simulink model "sowavedec2imaq"  (R2012a)
settings: Solver=FixedStepDiscrete  StartTime=0.0  StopTime=inf  RelTol=1e-3
undefined symbols (not defined in the file or in its folder): jet, none, videoinput
libraries: imaqlib x1, visionsinks x1
settings Model: ExtModeTrigDuration=100  Creator=harashin  LastModifiedBy=Shogo
settings DataIOCC: LimitDataPoints=on  SaveFormat=Array  ReturnWorkspaceOutputs=off
settings OptimizationCC: ExpressionDepthLimit=2147483647  OptimizeModelRefInitCode=on  LifeSpan=1  SimCompilerOptimization=Off
settings DebuggingCC: UnderspecifiedInitializationDetection=Classic  MergeDetectMultiDrivingBlocksExec=none  FcnCallInpInsideContextMsg=Enable All  FrameProcessingCompatibilityMsg=warning  StateNameClashWarn=warning  StrictBusMsg=Warning  SFUnexpectedBacktrackingDiag=warning  SFNoUnconditionalDefaultTransitionDiag=warning
settings HardwareCC: ProdBitPerPointer=32  ProdLargestAtomicInteger=Long  ProdLargestAtomicFloat=Double  ProdIntDivRoundTo=Undefined  ProdWordSize=32  ProdHWDeviceType=ARM Compatible->ARM Cortex
settings ModelReferenceCC: PropagateSignalLabelsOutOfModel=off
settings SFSimCC: SimUseLocalCustomCode=off
settings RTWCC: SystemTargetFile=realtime.tlc  GenerateMakefile=off  TemplateMakefile=realtime.tmf  Description=Real-Time Toolbox  RTWVerbose=off  ProcessScript=realtime_make_rtw_hook  RTWUseLocalCustomCode=off  RTWCompilerOptimization=Off
settings CodeAppCC: CustomSymbolStrType=$N$R$M
settings STFCustomTargetCC: TargetLibSuffix=.a  CodeReplacementLibrary=ANSI_C  GenerateSampleERTMain=on  ERTCustomFileBanners=on  SupportNonInlinedSFcns=off  SupportVariableSizeSignals=on  GRTInterface=off  SystemTargetFile=realtime.tlc
settings ERTTargetCC: CodeReplacementLibrary=ANSI_C  MultiwordLength=2048  GenerateSampleERTMain=on  ParMdlRefBuildCompliant=off  CompOptLevelCompliant=off  ConcurrentExecutionCompliant=off  CombineOutputUpdateFcns=off  ERTFirstTimeCompliant=off  SupportContinuousTime=on  SupportVariableSizeSignals=on  ModelStepFunctionPrototypeControlCompliant=off  CPPClassGenCompliant=off  ExtModeMexArgs='192.168.111.22' 0 17725  InlinedParameterPlacement=NonHierarchical  ERTSrcFileBannerTemplate=realtime_code_template.cgt  ERTHdrFileBannerTemplate=realtime_code_template.cgt  ERTDataSrcFileTemplate=realtime_code_template.cgt  ERTDataHdrFileTemplate=realtime_code_template.cgt  ERTCustomFileTemplate=realtime_file_process.tlc  ConvertIfToSwitch=off  SuppressUnreachableDefaultCases=off  MemSecPackage=Simulink

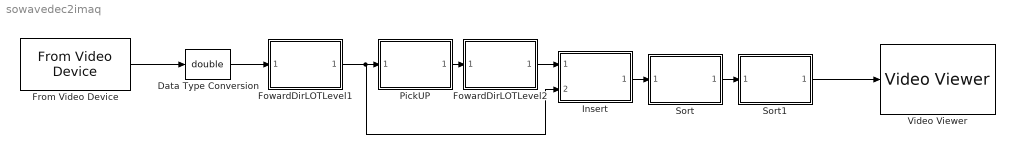
== system sowavedec2imaq ==
  Data Type Conversion : DataTypeConversion  OutDataTypeStr=double
  FowardDirLOTLevel1 : MATLAB Function  TreatAsAtomicUnit=on
      settings: PermitHierarchicalResolution=ParametersOnly
  FowardDirLOTLevel2 : MATLAB Function  TreatAsAtomicUnit=on
      settings: PermitHierarchicalResolution=ParametersOnly
  From Video Device : imaqlib/From Video Device  DeviceMenu=winvideo 1 (USB HD Webcam)  Device=winvideo 1 (Logicool HD Pro Webcam C920)  ObjConstructor=videoinput('winvideo', 1)  VideoFormatMenu=MJPG_1280x720  VideoFormat=I420_640x480  VideoSource=input1  ROIPosition=[0 0 480 640]  EnableHWTrigger=off  TriggerConfiguration=none/none  SampleTime=1/30  OutputPortsMode=One multidimensional signal  DataType=single  CanDoHWTrigger=no  ReturnedColorSpace=grayscale  BlockHandle=26.0013  ROIWidth=640  ROIHeight=480  ROIColumn=0  ROIRow=0  EngXMLPath=C:\Program Files\MATLAB\R2013a\toolbox\imaq\imaq\private  DevXMLPath=C:\Program Files\MATLAB\R2013a\toolbox\imaq\imaqadaptors\win64  EngLibPath=C:\Program Files\MATLAB\R2013a\toolbox\imaq\imaqblks\imaqmex\win64  ColorSpace=grayscale  BayerSensorAlignment=grbg
  Insert : MATLAB Function  TreatAsAtomicUnit=on
      settings: PermitHierarchicalResolution=ParametersOnly
  PickUP : MATLAB Function  TreatAsAtomicUnit=on
      settings: PermitHierarchicalResolution=ParametersOnly
  Sort : MATLAB Function  TreatAsAtomicUnit=on
      settings: PermitHierarchicalResolution=ParametersOnly
  Sort1 : MATLAB Function  TreatAsAtomicUnit=on
      settings: PermitHierarchicalResolution=ParametersOnly
  Video Viewer : visionsinks/Video Viewer  inputType=Obsolete7b  imagePorts=One multidimensional signal  useColorMap=off  colormapValue=jet(256)  specRange=off  minInputVal=0  maxInputVal=255  FigPos=[339 662 689 559]  AxisZoom=on  trueSizedOnce=off  OpenAtMdlStart=on
  wires:
  From Video Device/1 -> Data Type Conversion/1
  Sort1/1(coefActual) -> Video Viewer/1
  FowardDirLOTLevel1/1(coefActual) -> Insert/2(srcImg2), PickUP/1(srcImg)
  Data Type Conversion/1 -> FowardDirLOTLevel1/1(srcImg)
  PickUP/1(coefActual) -> FowardDirLOTLevel2/1(srcImg)
  FowardDirLOTLevel2/1(coefActual) -> Insert/1(srcImg1)
  Insert/1(coefActual) -> Sort/1(srcImg)
  Sort/1(coefActual) -> Sort1/1(srcImg)

== matlab function sowavedec2imaq/PickUP ==
  data: srcImg input; coefActual output
function coefActual = fcn(srcImg) %#codegen
%[ coefActual ] = coefPickUp(srcImg);
persistent hp;

if isempty(hp)
    
    % Instantiation
    hp = PickUp();
end

% Actual values
coefActual = step(hp,srcImg);

== matlab function sowavedec2imaq/FowardDirLOTLevel1 ==
  data: srcImg input; coefActual output
function coefActual = fcn(srcImg) %#codegen 
%[ coefActual ] = forwardDirLot(srcImg);
persistent hf;
if isempty(hf)
    % Instantiation
    hf = ForwardDirLotEmb();
end
% Actual values
coefActual = step(hf,srcImg);

== matlab function sowavedec2imaq/FowardDirLOTLevel2 ==
  data: srcImg input; coefActual output
function coefActual = fcn(srcImg) %#codegen
%[ coefActual ] = forwardDirLot(srcImg);
persistent hf;
if isempty(hf)
    % Instantiation
    hf = ForwardDirLotEmb();
end
% Actual values
coefActual = step(hf,srcImg);

== matlab function sowavedec2imaq/Insert ==
  data: srcImg1 input; coefActual output; srcImg2 input
function coefActual = fcn(srcImg1,srcImg2) %#codegen
%[ coefActual ] = coefInsert(srcImg1,srcImg2);
persistent hi;

if isempty(hi)
    % Instantiation
    hi = Insert();
end

% Actual values
coefActual = step(hi,srcImg1,srcImg2);

== matlab function sowavedec2imaq/Sort ==
  data: srcImg input; coefActual output
function coefActual = fcn(srcImg) %#codegen
%coefActual = SortCall(srcImg);
persistent hs;
if isempty(hs)
    % Instantiation
    hs = Sort();
end
% Actual values
coefActual = step(hs,srcImg);

== matlab function sowavedec2imaq/Sort1 ==
  data: srcImg input; coefActual output
function coefActual = fcn(srcImg) %#codegen
persistent hs;
if isempty(hs)
    % Instantiation
    hs = Sort();
end

[nRows, nCols] = size(srcImg);
coefLL = srcImg(1:nRows/2,1:nCols/2);
%afterSortLL = SortCall(coefLL);
afterSortLL = step(hs,coefLL);

srcImg(1:nRows/2,1:nCols/2) = afterSortLL;

srcImg2 = zeros(nRows,nCols);
srcImg2(1:nRows/4,1:nCols/4) = srcImg(1:nRows/4,1:nCols/4)*0.3;
srcImg2(nRows/4+1:nRows/2,1:nCols/4) = srcImg(nRows/4+1:nRows/2,1:nCols/4)*4;
srcImg2(1:nRows/4,nCols/4+1:nCols/2) = srcImg(1:nRows/4,nCols/4+1:nCols/2)*4;
srcImg2(nRows/4+1:nRows/2,nCols/4+1:nCols/2) = ...
    srcImg(nRows/4+1:nRows/2,nCols/4+1:nCols/2)*4;
srcImg2(nRows/2+1:nRows,1:nCols/2) = srcImg(nRows/2+1:nRows,1:nCols/2)*6;
srcImg2(1:nRows/2,nCols/2+1:nCols) = srcImg(1:nRows/2,nCols/2+1:nCols)*6;
srcImg2(nRows/2+1:nRows,nCols/2+1:nCols) = ...
    srcImg(nRows/2+1:nRows,nCols/2+1:nCols)*6;


coefActual = srcImg2;
